simulink model "GVCU_HIL_simscape"  (R2026a)
settings: Solver=ode3  StartTime=0  StopTime=10  FixedStep=0.001
model workspace (MAT data in the model file):
  CANoelibParameters : object (value not decoded)
values from neighbouring files (symbols this model uses):
  acc_pedal_data = pedal_data.accelerator_pedal_position_t0    [Init_Simscape_main.m]
  acc_pedal_time = pedal_data.t0    [Init_Simscape_main.m]
  brk_pedal_data = brake_pedal_data.shared_brakes_drvrBrkPedlPerc_t0    [Init_Simscape_main.m]
  brk_pedal_time = brake_pedal_data.t0    [Init_Simscape_main.m]
  cycle_len = zeros(1, num_cycles)    [Init_Simscape_main.m]
  cycle_speed_matrix = zeros(max_cycle_len, num_cycles)    [Init_Simscape_main.m]
  cycle_time_matrix = zeros(max_cycle_len, num_cycles)    [Init_Simscape_main.m]
  veh_speed_data = speed_data.shared_dynamicsVso_vehVelLgt_t0    [Init_Simscape_main.m]
  veh_speed_time = speed_data.t0    [Init_Simscape_main.m]
undefined symbols (not defined in the file or in its folder): Active, aero, AuxActive, bat, brake, config, environment, FL, FL_prs_voltage, FR, FR_prs_voltage, front, pos, powertrain, rear, RL, RL_prs_voltage, RR, RR_prs_voltage, tir, veh, VGetRawValueFlag, Voltage, VT2816_1_Ch1, VT2816_1_Ch2, VT2816_1_Ch3, VT2816_1_Ch4, VT2816_3_Ch13, VT2816_3_Ch14, VT7101_1_Out2, VTS, X, Y, Z
libraries: sm_lib x358, fl_lib x272, nesl_utility x193, canoelib x127, sdl_lib x36, autolibsharedcoupling x21, autolibcoupling x9, slpidlib x7, simulink x3, autolibshareddiff x3, autolibshared x3, autolibutils x1
(part 9 of 17)

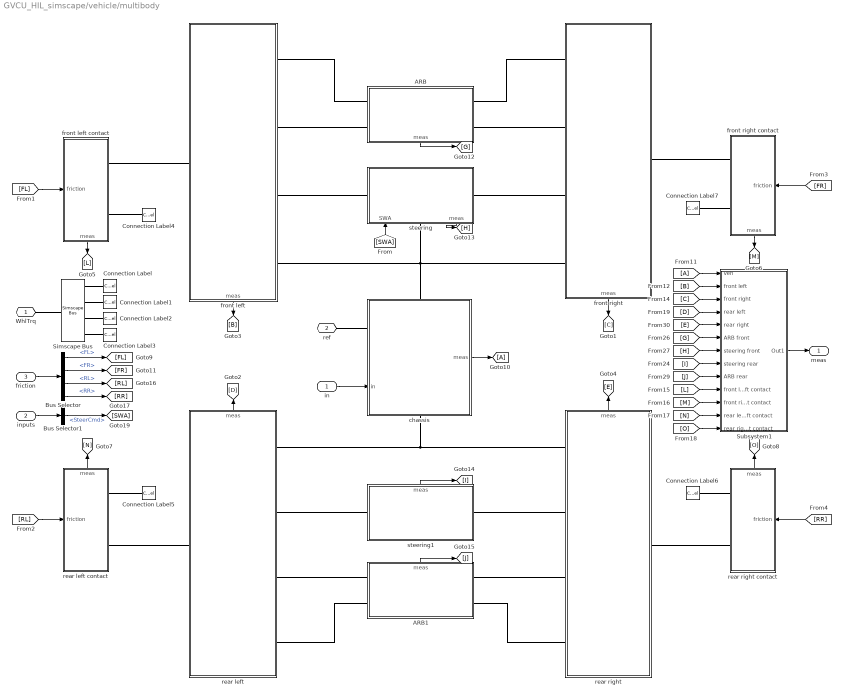
== system GVCU_HIL_simscape/vehicle/multibody ==
  in : Inport
  inputs : Inport  Port=2
  friction : Inport  Port=3
  ARB : Subsystem
      settings: PortSchema="{\"entries\":[{\"content\":{\"sides\":[{\"content\":{\"connectorIds\":[\"LConn1\",\"LConn2\"]},\"type\":\"ConnectorPlacement.EquallySpacedRectSide\",\"uuid\":\"44b83d78-7117-4f50-a128-c40c6db0e005\"},{\"content\":{\"connectorIds\":[\"RConn1\",\"RConn2\"],\"side\":\"RIGHT\"},\"type\":\"ConnectorPlacement.EquallySpacedRectSide\",\"uuid\":\"dcc56467-eb52-44b2-a421-ed24436307ce\"},{\"content\":{\"side\":\"TOP\"},\"type\":\"ConnectorPlacement.EquallySpacedRectSide\",\"uuid\":\"66a42ba5-e53f-479b-a6ea-7e29dc8adaf6\"},{\"content\":{\"connectorIds\":[\"Out1\"],\"side\":\"BOTTOM\"},\"type\":\"ConnectorPlacement.EquallySpacedRectSide\",\"uuid\":\"e20d4be4-d4bb-4d26-9635-b654396fd56f\"}]},\"type\":\"ConnectorPlacement.EquallySpacedConnector\",\"uuid\":\"7509cb20-f578-40f8-ba61-999a8824cfe4\"}],\"packageUris\":[\"http://schema.mathworks.com/mf0/Connector/R2020b\"],\"version\":\"1.0\"}"
  ARB1 : Subsystem
      settings: PortSchema="{\"entries\":[{\"content\":{\"sides\":[{\"content\":{\"connectorIds\":[\"LConn1\",\"LConn2\"]},\"type\":\"ConnectorPlacement.EquallySpacedRectSide\",\"uuid\":\"44b83d78-7117-4f50-a128-c40c6db0e005\"},{\"content\":{\"connectorIds\":[\"RConn1\",\"RConn2\"],\"side\":\"RIGHT\"},\"type\":\"ConnectorPlacement.EquallySpacedRectSide\",\"uuid\":\"dcc56467-eb52-44b2-a421-ed24436307ce\"},{\"content\":{\"connectorIds\":[\"Out1\"],\"side\":\"TOP\"},\"type\":\"ConnectorPlacement.EquallySpacedRectSide\",\"uuid\":\"66a42ba5-e53f-479b-a6ea-7e29dc8adaf6\"}]},\"type\":\"ConnectorPlacement.EquallySpacedConnector\",\"uuid\":\"7509cb20-f578-40f8-ba61-999a8824cfe4\"}],\"packageUris\":[\"http://schema.mathworks.com/mf0/Connector/R2020b\"],\"version\":\"1.0\"}"
  Bus Selector : BusSelector  OutputSignals=FL,FR,RL,RR
  Bus Selector1 : BusSelector  OutputSignals=SteerCmd
  Connection Label : ConnectionLabel  Label=FL
  Connection Label1 : ConnectionLabel  Label=FR
  Connection Label2 : ConnectionLabel  Label=RL
  Connection Label3 : ConnectionLabel  Label=RR
  Connection Label4 : ConnectionLabel  Label=FL
  Connection Label5 : ConnectionLabel  Label=RL
  Connection Label6 : ConnectionLabel  Label=RR
  Connection Label7 : ConnectionLabel  Label=FR
  From11 : From
  Goto10 : Goto
  Simscape Bus : SimscapeBus  HierarchyStrings=FL;FR;RL;RR
  Subsystem1 : Subsystem
  chassis : Subsystem
      settings: PortSchema="{\"entries\":[{\"content\":{\"sides\":[{\"content\":{\"connectorIds\":[\"LConn1\",\"In1\"]},\"type\":\"ConnectorPlacement.EquallySpacedRectSide\",\"uuid\":\"c24a0a87-e96f-44b7-bb9d-4d54604155f4\"},{\"content\":{\"connectorIds\":[\"Out1\"],\"side\":\"RIGHT\"},\"type\":\"ConnectorPlacement.EquallySpacedRectSide\",\"uuid\":\"a7cb0370-4bed-448c-a8ed-597510355169\"},{\"content\":{\"connectorIds\":[\"LConn2\"],\"side\":\"TOP\"},\"type\":\"ConnectorPlacement.EquallySpacedRectSide\",\"uuid\":\"f3c52e5d-562f-4591-a778-2d78a942b9f8\"},{\"content\":{\"connectorIds\":[\"RConn1\"],\"side\":\"BOTTOM\"},\"type\":\"ConnectorPlacement.EquallySpacedRectSide\",\"uuid\":\"7ef3619e-825e-48e3-8fdb-b0e1b2ee4c3a\"}]},\"type\":\"ConnectorPlacement.EquallySpacedConnector\",\"uuid\":\"67b61cb1-688b-4fcf-aa15-016bbf82641a\"}],\"packageUris\":[\"http://schema.mathworks.com/mf0/Connector/R2020b\"],\"version\":\"1.0\"}"
  front left : Subsystem
      settings: PortSchema="{\"entries\":[{\"content\":{\"sides\":[{\"content\":{\"connectorIds\":[\"LConn1\"]},\"type\":\"ConnectorPlacement.EquallySpacedRectSide\",\"uuid\":\"19de201b-0d55-468b-9ae9-f040ed0ebaa1\"},{\"content\":{\"connectorIds\":[\"RConn1\",\"RConn2\",\"RConn3\",\"RConn4\"],\"side\":\"RIGHT\"},\"type\":\"ConnectorPlacement.EquallySpacedRectSide\",\"uuid\":\"0a313072-8af5-469b-b8e4-48bb708ad821\"},{\"content\":{\"side\":\"TOP\"},\"type\":\"ConnectorPlacement.EquallySpacedRectSide\",\"uuid\":\"5fa73a83-add4-41d1-8bf2-6e1c7ef44456\"},{\"content\":{\"connectorIds\":[\"Out1\"],\"side\":\"BOTTOM\"},\"type\":\"ConnectorPlacement.EquallySpacedRectSide\",\"uuid\":\"99aac4ff-0e91-4277-96be-b0211bbbd05e\"}]},\"type\":\"ConnectorPlacement.EquallySpacedConnector\",\"uuid\":\"0106dc40-6661-4c74-95ab-8e6f8c5e0ff4\"}],\"packageUris\":[\"http://schema.mathworks.com/mf0/Connector/R2020b\"],\"version\":\"1.0\"}"
  front left contact : Subsystem
      settings: PortSchema="{\"entries\":[{\"content\":{\"sides\":[{\"content\":{\"connectorIds\":[\"In1\"]},\"type\":\"ConnectorPlacement.EquallySpacedRectSide\",\"uuid\":\"10158845-5afa-461c-a22d-1b912d59afd1\"},{\"content\":{\"connectorIds\":[\"RConn1\",\"RConn2\"],\"side\":\"RIGHT\"},\"type\":\"ConnectorPlacement.EquallySpacedRectSide\",\"uuid\":\"d8f36145-e6de-4ff7-929e-d1b9d10fe783\"},{\"content\":{\"side\":\"TOP\"},\"type\":\"ConnectorPlacement.EquallySpacedRectSide\",\"uuid\":\"7f3dfbca-e54d-431a-ba74-3f88cb4ee578\"},{\"content\":{\"connectorIds\":[\"Out1\"],\"side\":\"BOTTOM\"},\"type\":\"ConnectorPlacement.EquallySpacedRectSide\",\"uuid\":\"2d75498b-d206-48f5-8aff-45cacbfc615a\"}]},\"type\":\"ConnectorPlacement.EquallySpacedConnector\",\"uuid\":\"094a29d2-4f54-4ab7-b7e4-df405ec9cb17\"}],\"packageUris\":[\"http://schema.mathworks.com/mf0/Connector/R2020b\"],\"version\":\"1.0\"}"
  front right : Subsystem
      settings: PortSchema="{\"entries\":[{\"content\":{\"sides\":[{\"content\":{\"connectorIds\":[\"LConn1\",\"LConn2\",\"LConn3\",\"LConn4\"]},\"type\":\"ConnectorPlacement.EquallySpacedRectSide\",\"uuid\":\"1e088fd9-3d93-474e-8fe9-197185a633cf\"},{\"content\":{\"connectorIds\":[\"RConn1\"],\"side\":\"RIGHT\"},\"type\":\"ConnectorPlacement.EquallySpacedRectSide\",\"uuid\":\"782d0377-23b5-4dfd-8ac7-d3568aae0714\"},{\"content\":{\"side\":\"TOP\"},\"type\":\"ConnectorPlacement.EquallySpacedRectSide\",\"uuid\":\"3962e876-5f8e-408b-8e08-ce800b05363f\"},{\"content\":{\"connectorIds\":[\"Out1\"],\"side\":\"BOTTOM\"},\"type\":\"ConnectorPlacement.EquallySpacedRectSide\",\"uuid\":\"745efcfe-4536-4516-bf5a-c30453ee72e3\"}]},\"type\":\"ConnectorPlacement.EquallySpacedConnector\",\"uuid\":\"ffd119f6-ad19-4d62-b08f-fd8048e53da0\"}],\"packageUris\":[\"http://schema.mathworks.com/mf0/Connector/R2020b\"],\"version\":\"1.0\"}"
  front right contact : Subsystem
      settings: PortSchema="{\"entries\":[{\"content\":{\"sides\":[{\"content\":{\"connectorIds\":[\"In1\"]},\"type\":\"ConnectorPlacement.EquallySpacedRectSide\",\"uuid\":\"366ed39c-e506-485f-aedc-43f3a008ee89\"},{\"content\":{\"connectorIds\":[\"RConn1\",\"RConn2\"],\"side\":\"RIGHT\"},\"type\":\"ConnectorPlacement.EquallySpacedRectSide\",\"uuid\":\"70a828f7-7299-4f1a-95a3-d8e7b8390954\"},{\"content\":{\"connectorIds\":[\"Out1\"],\"side\":\"TOP\"},\"type\":\"ConnectorPlacement.EquallySpacedRectSide\",\"uuid\":\"0ab3354d-2824-40db-aebc-c093b7d793d8\"}]},\"type\":\"ConnectorPlacement.EquallySpacedConnector\",\"uuid\":\"4490982e-7f0c-4997-9546-ef978a19b2a8\"}],\"packageUris\":[\"http://schema.mathworks.com/mf0/Connector/R2020b\"],\"version\":\"1.0\"}"
  rear left : Subsystem
      settings: PortSchema="{\"entries\":[{\"content\":{\"sides\":[{\"content\":{\"connectorIds\":[\"LConn1\"]},\"type\":\"ConnectorPlacement.EquallySpacedRectSide\",\"uuid\":\"99636ad2-3001-422b-8269-7f0afa543239\"},{\"content\":{\"connectorIds\":[\"RConn1\",\"RConn2\",\"RConn3\",\"RConn4\"],\"side\":\"RIGHT\"},\"type\":\"ConnectorPlacement.EquallySpacedRectSide\",\"uuid\":\"6caf7980-c550-4646-898e-a2e6d571860b\"},{\"content\":{\"connectorIds\":[\"Out1\"],\"side\":\"TOP\"},\"type\":\"ConnectorPlacement.EquallySpacedRectSide\",\"uuid\":\"53eccbec-cba9-4e03-a09a-c4bd8c593235\"},{\"content\":{\"side\":\"BOTTOM\"},\"type\":\"ConnectorPlacement.EquallySpacedRectSide\",\"uuid\":\"e369446d-0d30-47ff-9006-d12c8ecdecf9\"}]},\"type\":\"ConnectorPlacement.EquallySpacedConnector\",\"uuid\":\"292a83a5-3a3e-4909-8366-ad11964dade1\"}],\"packageUris\":[\"http://schema.mathworks.com/mf0/Connector/R2020b\"],\"version\":\"1.0\"}"
  rear left contact : Subsystem
      settings: PortSchema="{\"entries\":[{\"content\":{\"sides\":[{\"content\":{\"connectorIds\":[\"In1\"]},\"type\":\"ConnectorPlacement.EquallySpacedRectSide\",\"uuid\":\"10158845-5afa-461c-a22d-1b912d59afd1\"},{\"content\":{\"connectorIds\":[\"RConn1\",\"RConn2\"],\"side\":\"RIGHT\"},\"type\":\"ConnectorPlacement.EquallySpacedRectSide\",\"uuid\":\"d8f36145-e6de-4ff7-929e-d1b9d10fe783\"},{\"content\":{\"connectorIds\":[\"Out1\"],\"side\":\"TOP\"},\"type\":\"ConnectorPlacement.EquallySpacedRectSide\",\"uuid\":\"7f3dfbca-e54d-431a-ba74-3f88cb4ee578\"}]},\"type\":\"ConnectorPlacement.EquallySpacedConnector\",\"uuid\":\"094a29d2-4f54-4ab7-b7e4-df405ec9cb17\"}],\"packageUris\":[\"http://schema.mathworks.com/mf0/Connector/R2020b\"],\"version\":\"1.0\"}"
  rear right : Subsystem
      settings: PortSchema="{\"entries\":[{\"content\":{\"sides\":[{\"content\":{\"connectorIds\":[\"LConn1\",\"LConn2\",\"LConn3\",\"LConn4\"]},\"type\":\"ConnectorPlacement.EquallySpacedRectSide\",\"uuid\":\"97554ec7-9fc3-491f-8a72-eaeb56dc13e3\"},{\"content\":{\"connectorIds\":[\"RConn1\"],\"side\":\"RIGHT\"},\"type\":\"ConnectorPlacement.EquallySpacedRectSide\",\"uuid\":\"01e3ceb2-8653-48cc-8018-c9fa0765a906\"},{\"content\":{\"connectorIds\":[\"Out1\"],\"side\":\"TOP\"},\"type\":\"ConnectorPlacement.EquallySpacedRectSide\",\"uuid\":\"f66f365d-d7f1-473b-ac81-c34d456abf41\"}]},\"type\":\"ConnectorPlacement.EquallySpacedConnector\",\"uuid\":\"3daf5b58-372f-4a47-a824-31f905f9d0f6\"}],\"packageUris\":[\"http://schema.mathworks.com/mf0/Connector/R2020b\"],\"version\":\"1.0\"}"
  rear right contact : Subsystem
      settings: PortSchema="{\"entries\":[{\"content\":{\"sides\":[{\"content\":{\"connectorIds\":[\"LConn1\",\"LConn2\"]},\"type\":\"ConnectorPlacement.EquallySpacedRectSide\",\"uuid\":\"50c969ea-b4f9-4e95-a8d7-0439ee002930\"},{\"content\":{\"connectorIds\":[\"In1\"],\"side\":\"RIGHT\"},\"type\":\"ConnectorPlacement.EquallySpacedRectSide\",\"uuid\":\"21bba6f4-d340-4ba8-8ff8-cca6003000cc\"},{\"content\":{\"connectorIds\":[\"Out1\"],\"side\":\"TOP\"},\"type\":\"ConnectorPlacement.EquallySpacedRectSide\",\"uuid\":\"17e17638-e1d3-4216-888f-e3f212538333\"}]},\"type\":\"ConnectorPlacement.EquallySpacedConnector\",\"uuid\":\"e91be55c-c97e-45e3-9316-75c991eef38b\"}],\"packageUris\":[\"http://schema.mathworks.com/mf0/Connector/R2020b\"],\"version\":\"1.0\"}"
  steering : Subsystem
      settings: PortSchema="{\"entries\":[{\"content\":{\"sides\":[{\"content\":{\"connectorIds\":[\"LConn1\"]},\"type\":\"ConnectorPlacement.EquallySpacedRectSide\",\"uuid\":\"8d82ea5c-1bae-45fe-ac82-53123a9b3f5e\"},{\"content\":{\"connectorIds\":[\"RConn1\"],\"side\":\"RIGHT\"},\"type\":\"ConnectorPlacement.EquallySpacedRectSide\",\"uuid\":\"e2db56e2-8468-453e-a935-2b5d90d5c02e\"},{\"content\":{\"side\":\"TOP\"},\"type\":\"ConnectorPlacement.EquallySpacedRectSide\",\"uuid\":\"66f010a1-1264-4266-a794-e542ee8c9be7\"},{\"content\":{\"connectorIds\":[\"In1\",\"RConn2\",\"Out1\"],\"side\":\"BOTTOM\"},\"type\":\"ConnectorPlacement.EquallySpacedRectSide\",\"uuid\":\"2ab87368-c822-4cdb-a3b2-bb1f2e0cbe7f\"}]},\"type\":\"ConnectorPlacement.EquallySpacedConnector\",\"uuid\":\"219c3897-806d-4045-90e2-26bf99ed85a1\"}],\"packageUris\":[\"http://schema.mathworks.com/mf0/Connector/R2020b\"],\"version\":\"1.0\"}"
  steering1 : Subsystem
      settings: PortSchema="{\"entries\":[{\"content\":{\"sides\":[{\"content\":{\"connectorIds\":[\"LConn1\"]},\"type\":\"ConnectorPlacement.EquallySpacedRectSide\",\"uuid\":\"fb5a7c7c-1f71-468f-8e2b-293f168c4d3f\"},{\"content\":{\"connectorIds\":[\"RConn1\"],\"side\":\"RIGHT\"},\"type\":\"ConnectorPlacement.EquallySpacedRectSide\",\"uuid\":\"5b9e4945-a95c-4a22-ad9b-f4b0b8937fba\"},{\"content\":{\"connectorIds\":[\"Out1\"],\"side\":\"TOP\"},\"type\":\"ConnectorPlacement.EquallySpacedRectSide\",\"uuid\":\"934bce12-3f30-409e-b265-a8a1cc310c4a\"}]},\"type\":\"ConnectorPlacement.EquallySpacedConnector\",\"uuid\":\"f5a21e72-9783-4a4e-b870-1cf7e777535b\"}],\"packageUris\":[\"http://schema.mathworks.com/mf0/Connector/R2020b\"],\"version\":\"1.0\"}"
  WhlTrq : PMIOPort  Side=Left
  ref : PMIOPort  Port=2  Side=Left
  meas : Outport
  wires:
  [SWA] -> steering/1(SWA)
  front left/1(meas) -> [B]
  rear right contact/1(meas) -> [O]
  rear left contact/1(meas) -> [N]
  front left contact/1(meas) -> [L]
  front right/1(meas) -> [C]
  rear left/1(meas) -> [D]
  front right contact/1(meas) -> [M]
  chassis/1(meas) -> Goto10/1
  rear right/1(meas) -> [E]
  Bus Selector1/1 -> [SWA]  "<SteerCmd>"
  inputs/1 -> Bus Selector1/1
  ARB/1(meas) -> [G]
  steering/1(meas) -> [H]
  steering1/1(meas) -> [I]
  ARB1/1(meas) -> [J]
  [B] -> Subsystem1/2(front left)
  [L] -> Subsystem1/10(front left contact)
  [C] -> Subsystem1/3(front right)
  [M] -> Subsystem1/11(front right contact)
  [G] -> Subsystem1/6(ARB front)
  [H] -> Subsystem1/7(steering front)
  [D] -> Subsystem1/4(rear left)
  [N] -> Subsystem1/12(rear left contact)
  [E] -> Subsystem1/5(rear right)
  [O] -> Subsystem1/13(rear right contact)
  [I] -> Subsystem1/8(steering rear)
  [J] -> Subsystem1/9(ARB rear)
  From11/1 -> Subsystem1/1(veh)
  Subsystem1/1(Out1) -> meas/1
  in/1 -> chassis/1(in)
  friction/1 -> Bus Selector/1
  Bus Selector/1 -> [FL]  "<FL>"
  Bus Selector/2 -> [FR]  "<FR>"
  Bus Selector/3 -> [RL]  "<RL>"
  Bus Selector/4 -> [RR]  "<RR>"
  [FL] -> front left contact/1(friction)
  [RL] -> rear left contact/1(friction)
  [FR] -> front right contact/1(friction)
  [RR] -> rear right contact/1(friction)
  connections:
  Connection Label7/LConn1 -- front right contact/RConn1
  ref/RConn1 -- chassis/LConn1
  ARB1/RConn2 -- rear right/LConn4
  rear left/RConn1 -- chassis/RConn1 -- rear right/LConn1
  front left/RConn4 -- steering/RConn2 -- front right/LConn4 -- chassis/LConn2
  Connection Label4/LConn1 -- front left contact/RConn2
  ARB/RConn1 -- front right/LConn1
  front left/RConn2 -- ARB/LConn2
  ARB/RConn2 -- front right/LConn2
  front right/RConn1 -- front right contact/RConn2
  steering/RConn1 -- front right/LConn3
  front left/RConn1 -- ARB/LConn1
  front left contact/RConn1 -- front left/LConn1
  rear right contact/LConn2 -- rear right/RConn1
  steering1/LConn1 -- rear left/RConn2
  rear left/RConn4 -- ARB1/LConn2
  rear left/RConn3 -- ARB1/LConn1
  rear right/LConn2 -- steering1/RConn1
  ARB1/RConn1 -- rear right/LConn3
  rear left contact/RConn2 -- rear left/LConn1
  Connection Label6/LConn1 -- rear right contact/LConn1
  steering/LConn1 -- front left/RConn3
  Connection Label5/LConn1 -- rear left contact/RConn1
  Simscape Bus/RConn1 -- WhlTrq/RConn1
  Connection Label/LConn1 -- Simscape Bus/LConn1
  Simscape Bus/LConn2 -- Connection Label1/LConn1
  Simscape Bus/LConn3 -- Connection Label2/LConn1
  Simscape Bus/LConn4 -- Connection Label3/LConn1

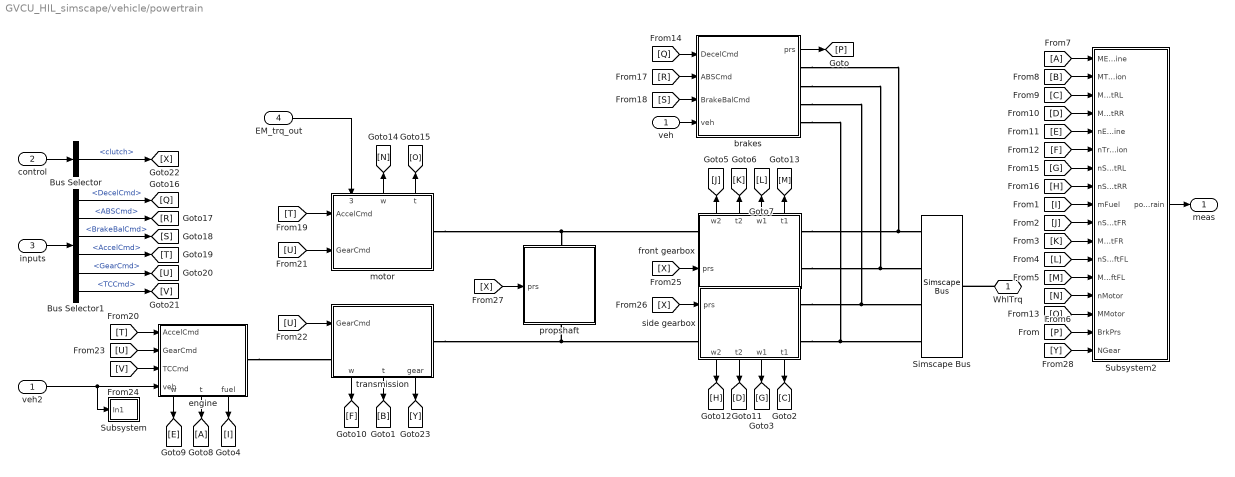
== system GVCU_HIL_simscape/vehicle/powertrain ==
  veh : Inport
  control : Inport  Port=2
  inputs : Inport  Port=3
  EM_trq_out : Inport  Port=4
  Bus Selector : BusSelector  OutputSignals=clutch
  Bus Selector1 : BusSelector  OutputSignals=DecelCmd,ABSCmd,BrakeBalCmd,AccelCmd,GearCmd,TCCmd
  From7 : From
  Goto8 : Goto
  Simscape Bus : SimscapeBus  HierarchyStrings=FL;FR;RL;RR
  Subsystem : Subsystem
  Subsystem2 : Subsystem
  brakes : Subsystem
  engine : Subsystem
      settings: PortSchema="{\"entries\":[{\"content\":{\"sides\":[{\"content\":{\"connectorIds\":[\"In1\",\"In2\",\"In3\",\"In4\"]},\"type\":\"ConnectorPlacement.EquallySpacedRectSide\",\"uuid\":\"a78e3356-1921-4efa-86ee-ec197aedbb96\"},{\"content\":{\"connectorIds\":[\"RConn1\"],\"side\":\"RIGHT\"},\"type\":\"ConnectorPlacement.EquallySpacedRectSide\",\"uuid\":\"41546e87-53dd-47be-ad0a-44218c6e7147\"},{\"content\":{\"side\":\"TOP\"},\"type\":\"ConnectorPlacement.EquallySpacedRectSide\",\"uuid\":\"0868fe6a-0ce7-41c0-87b1-c24c29d5bf2c\"},{\"content\":{\"connectorIds\":[\"Out1\",\"Out2\",\"Out3\"],\"side\":\"BOTTOM\"},\"type\":\"ConnectorPlacement.EquallySpacedRectSide\",\"uuid\":\"e86847d3-d00d-4616-b427-8230020483c2\"}]},\"type\":\"ConnectorPlacement.EquallySpacedConnector\",\"uuid\":\"338a52b8-b908-4274-bc1a-a3eae903fb18\"}],\"packageUris\":[\"http://schema.mathworks.com/mf0/Connector/R2020b\"],\"version\":\"1.0\"}"
  front gearbox : Subsystem
      settings: PortSchema="{\"entries\":[{\"content\":{\"sides\":[{\"content\":{\"connectorIds\":[\"LConn1\",\"In1\"]},\"type\":\"ConnectorPlacement.EquallySpacedRectSide\",\"uuid\":\"4b5bd540-f981-403d-a3c0-21cea5792707\"},{\"content\":{\"connectorIds\":[\"RConn1\",\"RConn2\"],\"side\":\"RIGHT\"},\"type\":\"ConnectorPlacement.EquallySpacedRectSide\",\"uuid\":\"db8e6c45-4440-4c46-8526-795a478301ab\"},{\"content\":{\"connectorIds\":[\"Out1\",\"Out2\",\"Out3\",\"Out4\"],\"side\":\"TOP\"},\"type\":\"ConnectorPlacement.EquallySpacedRectSide\",\"uuid\":\"3c4f3c49-5b91-4a57-ad94-4436adb36465\"}]},\"type\":\"ConnectorPlacement.EquallySpacedConnector\",\"uuid\":\"873cdc70-bb12-4c47-8236-9ecaebb66c28\"}],\"packageUris\":[\"http://schema.mathworks.com/mf0/Connector/R2020b\"],\"version\":\"1.0\"}"
  motor : Subsystem
      settings: PortSchema="{\"entries\":[{\"content\":{\"sides\":[{\"content\":{\"connectorIds\":[\"In1\",\"In2\"]},\"type\":\"ConnectorPlacement.EquallySpacedRectSide\",\"uuid\":\"8872ef77-aef5-44ab-bd09-c386537b6db6\"},{\"content\":{\"connectorIds\":[\"RConn1\"],\"side\":\"RIGHT\"},\"type\":\"ConnectorPlacement.EquallySpacedRectSide\",\"uuid\":\"8e814109-7cc3-4dbb-af0e-0bb3c3af015b\"},{\"content\":{\"connectorIds\":[\"In3\",\"Out1\",\"Out2\"],\"side\":\"TOP\"},\"type\":\"ConnectorPlacement.EquallySpacedRectSide\",\"uuid\":\"d6bbb977-d9f2-49ac-8838-af9f0d5a07e1\"}]},\"type\":\"ConnectorPlacement.EquallySpacedConnector\",\"uuid\":\"ff2df442-a81d-42d1-91a4-930a8e06f842\"}],\"packageUris\":[\"http://schema.mathworks.com/mf0/Connector/R2020b\"],\"version\":\"1.0\"}"
  propshaft : Subsystem
      settings: PortSchema="{\"entries\":[{\"content\":{\"sides\":[{\"content\":{\"connectorIds\":[\"In1\"]},\"type\":\"ConnectorPlacement.EquallySpacedRectSide\",\"uuid\":\"d74c70ba-453f-40cc-b257-82be2cfc77c8\"},{\"content\":{\"side\":\"RIGHT\"},\"type\":\"ConnectorPlacement.EquallySpacedRectSide\",\"uuid\":\"3ad33456-fba7-46bf-9dae-3669e8d1c7bf\"},{\"content\":{\"connectorIds\":[\"LConn1\"],\"side\":\"TOP\"},\"type\":\"ConnectorPlacement.EquallySpacedRectSide\",\"uuid\":\"e56339ea-fe76-4a6c-8c1f-8950ec15449d\"},{\"content\":{\"connectorIds\":[\"RConn1\"],\"side\":\"BOTTOM\"},\"type\":\"ConnectorPlacement.EquallySpacedRectSide\",\"uuid\":\"99006158-d2e6-44ab-b5b9-386e2116889a\"}]},\"type\":\"ConnectorPlacement.EquallySpacedConnector\",\"uuid\":\"1e2408ea-7505-408f-9d6e-80dc061e9f6e\"}],\"packageUris\":[\"http://schema.mathworks.com/mf0/Connector/R2020b\"],\"version\":\"1.0\"}"
  side gearbox : Subsystem
      settings: PortSchema="{\"entries\":[{\"content\":{\"sides\":[{\"content\":{\"connectorIds\":[\"In1\",\"LConn1\"]},\"type\":\"ConnectorPlacement.EquallySpacedRectSide\",\"uuid\":\"8c94453b-f679-4642-95d3-f9d99a2c2408\"},{\"content\":{\"connectorIds\":[\"RConn1\",\"RConn2\"],\"side\":\"RIGHT\"},\"type\":\"ConnectorPlacement.EquallySpacedRectSide\",\"uuid\":\"3bcbea54-e5b0-4650-b782-00c18ea383a7\"},{\"content\":{\"side\":\"TOP\"},\"type\":\"ConnectorPlacement.EquallySpacedRectSide\",\"uuid\":\"707a6b03-da98-480f-b93c-3d32e5658bd5\"},{\"content\":{\"connectorIds\":[\"Out1\",\"Out2\",\"Out3\",\"Out4\"],\"side\":\"BOTTOM\"},\"type\":\"ConnectorPlacement.EquallySpacedRectSide\",\"uuid\":\"a2021d0b-6ca2-49e7-9b1d-c01e0bfdef0d\"}]},\"type\":\"ConnectorPlacement.EquallySpacedConnector\",\"uuid\":\"d21a57c1-8b78-49d8-b9d2-27b607922f0d\"}],\"packageUris\":[\"http://schema.mathworks.com/mf0/Connector/R2020b\"],\"version\":\"1.0\"}"
  transmission : Subsystem
      settings: PortSchema="{\"entries\":[{\"content\":{\"sides\":[{\"content\":{\"connectorIds\":[\"In1\",\"LConn1\"]},\"type\":\"ConnectorPlacement.EquallySpacedRectSide\",\"uuid\":\"86e8cea5-b07c-40dd-bb6b-836fb2a21237\"},{\"content\":{\"connectorIds\":[\"RConn1\"],\"side\":\"RIGHT\"},\"type\":\"ConnectorPlacement.EquallySpacedRectSide\",\"uuid\":\"59522f78-d2d1-447e-be1e-cdc3e72ed8cb\"},{\"content\":{\"side\":\"TOP\"},\"type\":\"ConnectorPlacement.EquallySpacedRectSide\",\"uuid\":\"b992db60-f6d2-4879-b98d-54a12f763f72\"},{\"content\":{\"connectorIds\":[\"Out1\",\"Out2\",\"Out3\"],\"side\":\"BOTTOM\"},\"type\":\"ConnectorPlacement.EquallySpacedRectSide\",\"uuid\":\"d7b1bd10-aa14-42f4-8993-c98a02d1ca10\"}]},\"type\":\"ConnectorPlacement.EquallySpacedConnector\",\"uuid\":\"b24a2d83-8980-4644-9416-64d6e84609ca\"}],\"packageUris\":[\"http://schema.mathworks.com/mf0/Connector/R2020b\"],\"version\":\"1.0\"}"
  veh2 : InportShadow
  WhlTrq : PMIOPort  Side=Right
  meas : Outport
  wires:
  Bus Selector1/5 -> [U]  "<GearCmd>"
  inputs/1 -> Bus Selector1/1
  Bus Selector1/1 -> [Q]  "<DecelCmd>"
  Bus Selector1/4 -> [T]  "<AccelCmd>"
  engine/2(t) -> Goto8/1
  engine/1(w) -> [E]
  transmission/2(t) -> [B]
  transmission/1(w) -> [F]
  side gearbox/4(t1) -> [C]
  side gearbox/3(w1) -> [G]
  side gearbox/2(t2) -> [D]
  side gearbox/1(w2) -> [H]
  Bus Selector1/3 -> [S]  "<BrakeBalCmd>"
  veh/1 -> brakes/4(veh)
  Bus Selector1/2 -> [R]  "<ABSCmd>"
  Bus Selector1/6 -> [V]  "<TCCmd>"
  veh2/1 -> Subsystem/1(In1), engine/4(veh)
  From7/1 -> Subsystem2/1(MEngine)
  [B] -> Subsystem2/2(MTransmission)
  [C] -> Subsystem2/3(MSideShaftRL)
  [D] -> Subsystem2/4(MSideShaftRR)
  [E] -> Subsystem2/5(nEngine)
  [F] -> Subsystem2/6(nTransmission)
  [G] -> Subsystem2/7(nSideShaftRL)
  [H] -> Subsystem2/8(nSideShaftRR)
  Subsystem2/1(powertrain) -> meas/1
  engine/3(fuel) -> [I]
  [I] -> Subsystem2/9(mFuel)
  front gearbox/1(w2) -> [J]
  front gearbox/2(t2) -> [K]
  front gearbox/3(w1) -> [L]
  front gearbox/4(t1) -> [M]
  [M] -> Subsystem2/13(MSideShaftFL)
  [L] -> Subsystem2/12(nSideShaftFL)
  [K] -> Subsystem2/11(MSideShaftFR)
  [J] -> Subsystem2/10(nSIdeShaftFR)
  motor/1(w) -> [N]
  motor/2(t) -> [O]
  [N] -> Subsystem2/14(nMotor)
  [O] -> Subsystem2/15(MMotor)
  brakes/1(prs) -> [P]
  [P] -> Subsystem2/16(BrkPrs)
  [Q] -> brakes/1(DecelCmd)
  [R] -> brakes/2(ABSCmd)
  [S] -> brakes/3(BrakeBalCmd)
  [T] -> motor/1(AccelCmd)
  [T] -> engine/1(AccelCmd)
  [U] -> motor/2(GearCmd)
  [U] -> transmission/1(GearCmd)
  [U] -> engine/2(GearCmd)
  [V] -> engine/3(TCCmd)
  [X] -> front gearbox/1(prs)
  [X] -> side gearbox/1(prs)
  [X] -> propshaft/1(prs)
  control/1 -> Bus Selector/1
  Bus Selector/1 -> [X]  "<clutch>"
  transmission/3(gear) -> [Y]
  [Y] -> Subsystem2/17(NGear)
  EM_trq_out/1 -> motor/3(EM_trq_out)
  connections:
  brakes/RConn1 -- front gearbox/RConn1 -- Simscape Bus/LConn1
  brakes/RConn2 -- front gearbox/RConn2 -- Simscape Bus/LConn2
  engine/RConn1 -- transmission/LConn1
  side gearbox/RConn2 -- brakes/RConn4 -- Simscape Bus/LConn4
  side gearbox/RConn1 -- brakes/RConn3 -- Simscape Bus/LConn3
  transmission/RConn1 -- propshaft/RConn1 -- side gearbox/LConn1
  WhlTrq/RConn1 -- Simscape Bus/RConn1
  motor/RConn1 -- propshaft/LConn1 -- front gearbox/LConn1

== system GVCU_HIL_simscape/Driver/Driver/Dec_controller ==
  Vel_ref : Inport
  Vel_fdk : Inport  Port=2
  PI Controller : slpidlib/PID Controller  Controller=PI  Form=Parallel  TimeDomain=Discrete-time  UseExternalTs=off  SampleTime=-1  IntegratorMethod=Forward Euler  FilterMethod=Forward Euler  ControllerParametersSource=internal  P=1  I=1  UseKiTs=on  D=0  UseExternalDerivativeSource=off  N=100  UseFilter=on  TunerSelectOption=Transfer Function Based (PID Tuner App)  InitialConditionSource=internal  InitialConditionForIntegrator=0  InitialConditionForFilter=0  DifferentiatorICPrevScaledInput=0  ExternalReset=level  TrackingMode=off  Kt=1  LimitOutput=on  SatLimitsSource=internal  UpperSaturationLimit=50  LowerSaturationLimit=0  LinearizeAsGain=on  AntiWindupMode=clamping  Kb=1  LimitIntegrator=off  UpperIntegratorSaturationLimit=inf  LowerIntegratorSaturationLimit=-inf  RndMeth=Simplest  POutMin=[]  POutMax=[]  IOutMin=[]  IOutMax=[]  DOutMin=[]  DOutMax=[]  NOutMin=[]  NOutMax=[]  SumOutMin=[]  SumOutMax=[]  SaturationOutDataTypeStr=Inherit: Inherit via back propagation  SaturationOutMin=[]  SaturationOutMax=[]  PParamMin=[]  PParamMax=[]  IParamMin=[]  IParamMax=[]  DParamMin=[]  DParamMax=[]  NParamMin=[]  NParamMax=[]  KbParamMin=[]  KbParamMax=[]  KtParamMin=[]  KtParamMax=[]  KbOutMin=[]  KbOutMax=[]  KtOutMin=[]  KtOutMax=[]  IntegratorOutMin=[]  IntegratorOutMax=[]  FilterOutMin=[]  FilterOutMax=[]  SumI1OutMin=[]  SumI1OutMax=[]  SumI2OutMin=[]  SumI2OutMax=[]  SumI3OutMin=[]  SumI3OutMax=[]  SumI4OutMin=[]  SumI4OutMax=[]  SumDOutMin=[]  SumDOutMax=[]  DifferentiatorOutMin=[]  DifferentiatorOutMax=[]  FilterDiffOutCoefMin=[]  FilterDiffOutCoefMax=[]  ReciprocalOutMin=[]  ReciprocalOutMax=[]  SumDenOutMin=[]  SumDenOutMax=[]  SumNumOutMin=[]  SumNumOutMax=[]  DivideOutMin=[]  DivideOutMax=[]  UdiffTsProdOutMin=[]  UdiffTsProdOutMax=[]  NTsProdOutMin=[]  NTsProdOutMax=[]  UintegralTsProdOutMin=[]  UintegralTsProdOutMax=[]  UngainTsProdOutMin=[]  UngainTsProdOutMax=[]  ClampingZeroOutDataTypeStr=Inherit: Inherit via back propagation  ClampingZeroOutMin=[]  ClampingZeroOutMax=[]  FilterDenConstantOutDataTypeStr=Inherit: Inherit via back propagation  FilterDenConstantOutMin=[]  FilterDenConstantOutMax=[]  PCopyOutDataTypeStr=Inherit: Inherit via back propagation  PCopyOutMin=[]  PCopyOutMax=[]  NCopyOutDataTypeStr=Inherit: Inherit via back propagation  NCopyOutMin=[]  NCopyOutMax=[]  IntegratorContinuousStateAttributes=''  IntegratorStateMustResolveToSignalObject=off  IntegratorRTWStateStorageClass=Auto  FilterContinuousStateAttributes=''  FilterStateMustResolveToSignalObject=off  FilterRTWStateStorageClass=Auto  ParallelPVariant=InternalParameters  IdealPVariant=Disabled  IVariant=InternalParameters  DVariant=Disabled  IntegratorVariant=Discrete  SatVariant=Enabled  AWVariant=DiscClampingParallel  PCopyVariant=Disabled  TRVariant=Disabled  FdbkBlocksVariant=Forward  IdealPFdbkVariant=Disabled  SatFdbkVariant=Disabled  DerivativeFilterVariant=Disabled  NVariant=Disabled  NCopyVariant=Disabled_SignalSpec  FilterICVariant=Disabled  IntegratorICVariant=InternalICs  ExternalResetVariant=ExternalReset  TRSumVariant=Passthrough  SumFdbkVariant=Disabled  SumVariant=Sum_PI  TsampFilterVariant=InternalTs  TsampNgainVariant=Passthrough  TsampIntegralVariant=Disabled_SignalSpec  ExternalSaturationOutDataTypeStr=Inherit: Same as second input  DerivativeSourceVariant=Disabled  PreIntVariant=InternalPreInt
      settings: LibrarySourceBlock=mcbhdllib/Controls/Controllers/PI Controller
  Relay : Relay  OnSwitchValue=10  OffSwitchValue=1
  Subtract : Sum  Inputs=+-
  Dec_cmd : Outport
  wires:
  Vel_ref/1 -> Subtract/2
  Vel_fdk/1 -> Subtract/1
  PI Controller/1 -> Dec_cmd/1
  Subtract/1 -> PI Controller/1, Relay/1
  Relay/1 -> PI Controller/2

== system GVCU_HIL_simscape/Driver/Driver/LPF ==
  u : Inport
  Divide : Product  Inputs=/
  Error LPF : autolibutils/Cont LPF Dyn  aMode=aMode  dataType=off
  tauerr : Constant  Value=0.03  SampleTime=-1
  y : Outport  VectorParamsAs1DForOutWhenUnconnected=off
  wires:
  Error LPF/1 -> y/1
  Divide/1 -> Error LPF/2
  tauerr/1 -> Divide/1
  u/1 -> Error LPF/1

== system GVCU_HIL_simscape/GVCU - HiL/Commented messages/Message Output12 ==
  In1 : Inport
  Bus Selector : BusSelector  OutputSignals=e2e_alive_counter_disabled,e2e_checksum_disabled,e_motor_pump_fault,e_motor_pump_power_on,e_motor_pump_speed,e_motor_pump_warning,front_left_fan_fault,front_left_fan_power_on,front_left_fan_speed,front_left_fan_warning,hv_bat_pump_fault,hv_bat_pump_power_on,hv_bat_pump_speed,hv_bat_pump_warning
  S-Function_1 : S-Function  FunctionName=sigout  Parameters=dbName;nodeName;msgName;14;'e2e_alive_counter_disabled';'e2e_checksum_disabled';'e_motor_pump_fault';'e_motor_pump_power_on';'e_motor_pump_speed';'e_motor_pump_warning';'front_left_fan_fault';'front_left_fan_power_on';'front_left_fan_speed';'front_left_fan_warning';'hv_bat_pump_fault';'hv_bat_pump_power_on';'hv_bat_pump_speed';'hv_bat_pump_warning';VGetRawValueFlag(rawValue);'inherited'  SFunctionDeploymentMode=off  EnableBusSupport=off
      settings: AttributesFormatString=e2e_alive_counter_disabled\ne2e_checksum_disabled\ne_motor_pump_fault\ne_motor_pump_power_on\ne_motor_pump_speed\ne_motor_pump_warning\nfront_left_fan_fault\nfront_left_fan_power_on\nfront_left_fan_speed\nfront_left_fan_warning\nhv_bat_pump_fault\nhv_bat_pump_power_on\nhv_bat_pump_speed\nhv_bat_pump_warning\n
  wires:
  In1/1 -> Bus Selector/1
  Bus Selector/1 -> S-Function_1/1  "<e2e_alive_counter_disabled>"
  Bus Selector/2 -> S-Function_1/2  "<e2e_checksum_disabled>"
  Bus Selector/3 -> S-Function_1/3  "<e_motor_pump_fault>"
  Bus Selector/4 -> S-Function_1/4  "<e_motor_pump_power_on>"
  Bus Selector/5 -> S-Function_1/5  "<e_motor_pump_speed>"
  Bus Selector/6 -> S-Function_1/6  "<e_motor_pump_warning>"
  Bus Selector/7 -> S-Function_1/7  "<front_left_fan_fault>"
  Bus Selector/8 -> S-Function_1/8  "<front_left_fan_power_on>"
  Bus Selector/9 -> S-Function_1/9  "<front_left_fan_speed>"
  Bus Selector/10 -> S-Function_1/10  "<front_left_fan_warning>"
  Bus Selector/11 -> S-Function_1/11  "<hv_bat_pump_fault>"
  Bus Selector/12 -> S-Function_1/12  "<hv_bat_pump_power_on>"
  Bus Selector/13 -> S-Function_1/13  "<hv_bat_pump_speed>"
  Bus Selector/14 -> S-Function_1/14  "<hv_bat_pump_warning>"

== system GVCU_HIL_simscape/GVCU - HiL/Commented messages/Message Output13 ==
  In1 : Inport
  Bus Selector : BusSelector  OutputSignals=e2e_alive_counter_disabled,e2e_checksum_disabled,inverter_pump_fault,inverter_pump_power_on,inverter_pump_speed,inverter_pump_warning
  S-Function_1 : S-Function  FunctionName=sigout  Parameters=dbName;nodeName;msgName;6;'e2e_alive_counter_disabled';'e2e_checksum_disabled';'inverter_pump_fault';'inverter_pump_power_on';'inverter_pump_speed';'inverter_pump_warning';VGetRawValueFlag(rawValue);'inherited'  SFunctionDeploymentMode=off  EnableBusSupport=off
      settings: AttributesFormatString=e2e_alive_counter_disabled\ne2e_checksum_disabled\ninverter_pump_fault\ninverter_pump_power_on\ninverter_pump_speed\ninverter_pump_warning\n
  wires:
  In1/1 -> Bus Selector/1
  Bus Selector/1 -> S-Function_1/1  "<e2e_alive_counter_disabled>"
  Bus Selector/2 -> S-Function_1/2  "<e2e_checksum_disabled>"
  Bus Selector/3 -> S-Function_1/3  "<inverter_pump_fault>"
  Bus Selector/4 -> S-Function_1/4  "<inverter_pump_power_on>"
  Bus Selector/5 -> S-Function_1/5  "<inverter_pump_speed>"
  Bus Selector/6 -> S-Function_1/6  "<inverter_pump_warning>"

== system GVCU_HIL_simscape/GVCU - HiL/Commented messages/Message Output14 ==
  In1 : Inport
  Bus Selector : BusSelector  OutputSignals=u_lift_cyl_fl,u_lift_cyl_fr,u_wishbone_angle_fl,u_wishbone_angle_fr
  S-Function_1 : S-Function  FunctionName=sigout  Parameters=dbName;nodeName;msgName;4;'u_lift_cyl_fl';'u_lift_cyl_fr';'u_wishbone_angle_fl';'u_wishbone_angle_fr';VGetRawValueFlag(rawValue);'inherited'  SFunctionDeploymentMode=off  EnableBusSupport=off
      settings: AttributesFormatString=u_lift_cyl_fl\nu_lift_cyl_fr\nu_wishbone_angle_fl\nu_wishbone_angle_fr\n
  wires:
  In1/1 -> Bus Selector/1
  Bus Selector/1 -> S-Function_1/1  "<u_lift_cyl_fl>"
  Bus Selector/2 -> S-Function_1/2  "<u_lift_cyl_fr>"
  Bus Selector/3 -> S-Function_1/3  "<u_wishbone_angle_fl>"
  Bus Selector/4 -> S-Function_1/4  "<u_wishbone_angle_fr>"

== system GVCU_HIL_simscape/GVCU - HiL/Commented messages/Message Output15 ==
  In1 : Inport
  Bus Selector : BusSelector  OutputSignals=actv_re,snsr_data_rcl,snsr_data_rcr,snsr_data_rl,snsr_data_rll,snsr_data_rr,snsr_data_rrl,snsr_st_rcl,snsr_st_rcr,snsr_st_rl,snsr_st_rll,snsr_st_rr,snsr_st_rrl
  S-Function_1 : S-Function  FunctionName=sigout  Parameters=dbName;nodeName;msgName;13;'actv_re';'snsr_data_rcl';'snsr_data_rcr';'snsr_data_rl';'snsr_data_rll';'snsr_data_rr';'snsr_data_rrl';'snsr_st_rcl';'snsr_st_rcr';'snsr_st_rl';'snsr_st_rll';'snsr_st_rr';'snsr_st_rrl';VGetRawValueFlag(rawValue);'inherited'  SFunctionDeploymentMode=off  EnableBusSupport=off
      settings: AttributesFormatString=actv_re\nsnsr_data_rcl\nsnsr_data_rcr\nsnsr_data_rl\nsnsr_data_rll\nsnsr_data_rr\nsnsr_data_rrl\nsnsr_st_rcl\nsnsr_st_rcr\nsnsr_st_rl\nsnsr_st_rll\nsnsr_st_rr\nsnsr_st_rrl\n
  wires:
  In1/1 -> Bus Selector/1
  Bus Selector/1 -> S-Function_1/1  "<actv_re>"
  Bus Selector/2 -> S-Function_1/2  "<snsr_data_rcl>"
  Bus Selector/3 -> S-Function_1/3  "<snsr_data_rcr>"
  Bus Selector/4 -> S-Function_1/4  "<snsr_data_rl>"
  Bus Selector/5 -> S-Function_1/5  "<snsr_data_rll>"
  Bus Selector/6 -> S-Function_1/6  "<snsr_data_rr>"
  Bus Selector/7 -> S-Function_1/7  "<snsr_data_rrl>"
  Bus Selector/8 -> S-Function_1/8  "<snsr_st_rcl>"
  Bus Selector/9 -> S-Function_1/9  "<snsr_st_rcr>"
  Bus Selector/10 -> S-Function_1/10  "<snsr_st_rl>"
  Bus Selector/11 -> S-Function_1/11  "<snsr_st_rll>"
  Bus Selector/12 -> S-Function_1/12  "<snsr_st_rr>"
  Bus Selector/13 -> S-Function_1/13  "<snsr_st_rrl>"

== system GVCU_HIL_simscape/GVCU - HiL/Commented messages/Message Output16 ==
  In1 : Inport
  Bus Selector : BusSelector  OutputSignals=actv_frnt,snsr_data_fcl,snsr_data_fcr,snsr_data_fl,snsr_data_fll,snsr_data_fr,snsr_data_frl,snsr_st_fcl,snsr_st_fcr,snsr_st_fl,snsr_st_fll,snsr_st_fr,snsr_st_frl
  S-Function_1 : S-Function  FunctionName=sigout  Parameters=dbName;nodeName;msgName;13;'actv_frnt';'snsr_data_fcl';'snsr_data_fcr';'snsr_data_fl';'snsr_data_fll';'snsr_data_fr';'snsr_data_frl';'snsr_st_fcl';'snsr_st_fcr';'snsr_st_fl';'snsr_st_fll';'snsr_st_fr';'snsr_st_frl';VGetRawValueFlag(rawValue);'inherited'  SFunctionDeploymentMode=off  EnableBusSupport=off
      settings: AttributesFormatString=actv_frnt\nsnsr_data_fcl\nsnsr_data_fcr\nsnsr_data_fl\nsnsr_data_fll\nsnsr_data_fr\nsnsr_data_frl\nsnsr_st_fcl\nsnsr_st_fcr\nsnsr_st_fl\nsnsr_st_fll\nsnsr_st_fr\nsnsr_st_frl\n
  wires:
  In1/1 -> Bus Selector/1
  Bus Selector/1 -> S-Function_1/1  "<actv_frnt>"
  Bus Selector/2 -> S-Function_1/2  "<snsr_data_fcl>"
  Bus Selector/3 -> S-Function_1/3  "<snsr_data_fcr>"
  Bus Selector/4 -> S-Function_1/4  "<snsr_data_fl>"
  Bus Selector/5 -> S-Function_1/5  "<snsr_data_fll>"
  Bus Selector/6 -> S-Function_1/6  "<snsr_data_fr>"
  Bus Selector/7 -> S-Function_1/7  "<snsr_data_frl>"
  Bus Selector/8 -> S-Function_1/8  "<snsr_st_fcl>"
  Bus Selector/9 -> S-Function_1/9  "<snsr_st_fcr>"
  Bus Selector/10 -> S-Function_1/10  "<snsr_st_fl>"
  Bus Selector/11 -> S-Function_1/11  "<snsr_st_fll>"
  Bus Selector/12 -> S-Function_1/12  "<snsr_st_fr>"
  Bus Selector/13 -> S-Function_1/13  "<snsr_st_frl>"

== system GVCU_HIL_simscape/GVCU - HiL/Commented messages/Message Output2 ==
  In1 : Inport
  Bus Selector : BusSelector  OutputSignals=e2e_alive_counter_disabled,e2e_checksum_disabled,front_center_left_fan_fault,front_center_left_fan_power_on,front_center_left_fan_speed,front_center_left_fan_warning,front_center_right_fan_fault,front_center_right_fan_power_on,front_center_right_fan_speed,front_center_right_fan_warning,front_right_fan_fault,front_right_fan_power_on,front_right_fan_speed,front_right_fan_warning
  S-Function_1 : S-Function  FunctionName=sigout  Parameters=dbName;nodeName;msgName;14;'e2e_alive_counter_disabled';'e2e_checksum_disabled';'front_center_left_fan_fault';'front_center_left_fan_power_on';'front_center_left_fan_speed';'front_center_left_fan_warning';'front_center_right_fan_fault';'front_center_right_fan_power_on';'front_center_right_fan_speed';'front_center_right_fan_warning';'front_right_fan_fault';'front_right_fan_power_on';'front_right_fan_speed';'front_right_fan_warning';VGetRawValueFlag(rawValue);'inherited'  SFunctionDeploymentMode=off  EnableBusSupport=off
      settings: AttributesFormatString=e2e_alive_counter_disabled\ne2e_checksum_disabled\nfront_center_left_fan_fault\nfront_center_left_fan_power_on\nfront_center_left_fan_speed\nfront_center_left_fan_warning\nfront_center_right_fan_fault\nfront_center_right_fan_power_on\nfront_center_right_fan_speed\nfront_center_right_fan_warning\nfront_right_fan_fault\nfront_right_fan_power_on\nfront_right_fan_speed\nfront_right_fan_warning\n
  wires:
  In1/1 -> Bus Selector/1
  Bus Selector/1 -> S-Function_1/1  "<e2e_alive_counter_disabled>"
  Bus Selector/2 -> S-Function_1/2  "<e2e_checksum_disabled>"
  Bus Selector/3 -> S-Function_1/3  "<front_center_left_fan_fault>"
  Bus Selector/4 -> S-Function_1/4  "<front_center_left_fan_power_on>"
  Bus Selector/5 -> S-Function_1/5  "<front_center_left_fan_speed>"
  Bus Selector/6 -> S-Function_1/6  "<front_center_left_fan_warning>"
  Bus Selector/7 -> S-Function_1/7  "<front_center_right_fan_fault>"
  Bus Selector/8 -> S-Function_1/8  "<front_center_right_fan_power_on>"
  Bus Selector/9 -> S-Function_1/9  "<front_center_right_fan_speed>"
  Bus Selector/10 -> S-Function_1/10  "<front_center_right_fan_warning>"
  Bus Selector/11 -> S-Function_1/11  "<front_right_fan_fault>"
  Bus Selector/12 -> S-Function_1/12  "<front_right_fan_power_on>"
  Bus Selector/13 -> S-Function_1/13  "<front_right_fan_speed>"
  Bus Selector/14 -> S-Function_1/14  "<front_right_fan_warning>"

== system GVCU_HIL_simscape/GVCU - HiL/Commented messages/Message Output20 ==
  In1 : Inport
  Bus Selector : BusSelector  OutputSignals=E2eAliveCounter_Disable,E2eChecksum_Disable,acc_dft_actv_st,acc_dft_dist_lvl,auto_upsh_btn_st,drv_cfg_req,drv_st,esp_st_req,forced_chrg_btn_st,lift_mod_btn_st,man_mod_btn_st,suppg_mod_req,tire_mdl_req
  S-Function_1 : S-Function  FunctionName=sigout  Parameters=dbName;nodeName;msgName;13;'E2eAliveCounter_Disable';'E2eChecksum_Disable';'acc_dft_actv_st';'acc_dft_dist_lvl';'auto_upsh_btn_st';'drv_cfg_req';'drv_mod_req';'esp_st_req';'forced_chrg_btn_st';'lift_mod_btn_st';'man_mod_btn_st';'suppg_mod_req';'tire_mdl_req';VGetRawValueFlag(rawValue);'inherited'  SFunctionDeploymentMode=off  EnableBusSupport=off
      settings: AttributesFormatString=E2eAliveCounter_Disable\nE2eChecksum_Disable\nacc_dft_actv_st\nacc_dft_dist_lvl\nauto_upsh_btn_st\ndrv_cfg_req\ndrv_mod_req\nesp_st_req\nforced_chrg_btn_st\nlift_mod_btn_st\nman_mod_btn_st\nsuppg_mod_req\ntire_mdl_req\n
  wires:
  In1/1 -> Bus Selector/1
  Bus Selector/1 -> S-Function_1/1  "<E2eAliveCounter_Disable>"
  Bus Selector/2 -> S-Function_1/2  "<E2eChecksum_Disable>"
  Bus Selector/3 -> S-Function_1/3  "<acc_dft_actv_st>"
  Bus Selector/4 -> S-Function_1/4  "<acc_dft_dist_lvl>"
  Bus Selector/5 -> S-Function_1/5  "<auto_upsh_btn_st>"
  ? -> S-Function_1/6  "<drift_mod_st_req>"
  Bus Selector/6 -> S-Function_1/7  "<drv_cfg_req>"
  Bus Selector/7 -> S-Function_1/8  "<drv_st>"
  Bus Selector/8 -> S-Function_1/9  "<esp_st_req>"
  Bus Selector/9 -> S-Function_1/10  "<forced_chrg_btn_st>"
  Bus Selector/10 -> S-Function_1/11  "<lift_mod_btn_st>"
  Bus Selector/11 -> S-Function_1/12  "<man_mod_btn_st>"
  Bus Selector/13 -> S-Function_1/13  "<tire_mdl_req>"

== system GVCU_HIL_simscape/GVCU - HiL/Commented messages/Message Output4 ==
  In1 : Inport
  Bus Selector : BusSelector  OutputSignals=CrashSeverity,DriverSideCrash,E2eAliveCounter,E2eChecksum,FrontCrash,PassSideCrash,RearCrash,RolloverCrash
  S-Function_1 : S-Function  FunctionName=sigout  Parameters=dbName;nodeName;msgName;8;'CrashSeverity';'DriverSideCrash';'E2eAliveCounter';'E2eChecksum';'FrontCrash';'PassSideCrash';'RearCrash';'RolloverCrash';VGetRawValueFlag(rawValue);'inherited'  SFunctionDeploymentMode=off  EnableBusSupport=off
      settings: AttributesFormatString=CrashSeverity\nDriverSideCrash\nE2eAliveCounter\nE2eChecksum\nFrontCrash\nPassSideCrash\nRearCrash\nRolloverCrash\n
  wires:
  In1/1 -> Bus Selector/1
  Bus Selector/1 -> S-Function_1/1  "<CrashSeverity>"
  Bus Selector/2 -> S-Function_1/2  "<DriverSideCrash>"
  Bus Selector/3 -> S-Function_1/3  "<E2eAliveCounter>"
  Bus Selector/4 -> S-Function_1/4  "<E2eChecksum>"
  Bus Selector/5 -> S-Function_1/5  "<FrontCrash>"
  Bus Selector/6 -> S-Function_1/6  "<PassSideCrash>"
  Bus Selector/7 -> S-Function_1/7  "<RearCrash>"
  Bus Selector/8 -> S-Function_1/8  "<RolloverCrash>"

== system GVCU_HIL_simscape/GVCU - HiL/Commented messages/Message Output5 ==
  In1 : Inport
  Bus Selector : BusSelector  OutputSignals=CrashOutput,E2eAliveCounter,E2eChecksum
  S-Function_1 : S-Function  FunctionName=sigout  Parameters=dbName;nodeName;msgName;3;'CrashOutput';'E2eAliveCounter';'E2eChecksum';VGetRawValueFlag(rawValue);'inherited'  SFunctionDeploymentMode=off  EnableBusSupport=off
      settings: AttributesFormatString=CrashOutput\nE2eAliveCounter\nE2eChecksum\n
  wires:
  In1/1 -> Bus Selector/1
  Bus Selector/1 -> S-Function_1/1  "<CrashOutput>"
  Bus Selector/2 -> S-Function_1/2  "<E2eAliveCounter>"
  Bus Selector/3 -> S-Function_1/3  "<E2eChecksum>"

== system GVCU_HIL_simscape/GVCU - HiL/Commented messages/Message Output6 ==
  In1 : Inport
  Bus Selector : BusSelector  OutputSignals=center_left_fan_bat_vltg,center_left_fan_can_collision,center_left_fan_can_watchdog,center_left_fan_motor_stall,center_left_fan_over_crnt,center_left_fan_over_pwr,center_left_fan_over_temp,center_right_fan_bat_vltg,center_right_fan_can_collision,center_right_fan_can_watchdog,center_right_fan_motor_stall,center_right_fan_over_crnt,center_right_fan_over_pwr,center_right_fan_over_temp,e_mot_pump_comm_fault,e_mot_pump_int_op_fault,e_mot_pump_over_crnt,e_mot_pump_over_temp,e_mot_pump_vltg_err,front_left_fan_bat_vltg,front_left_fan_can_collision,front_left_fan_can_watchdog,front_left_fan_motor_stall,front_left_fan_over_crnt,front_left_fan_over_pwr,front_left_fan_over_temp,front_right_fan_bat_vltg,front_right_fan_can_collision,front_right_fan_can_watchdog,front_right_fan_motor_stall,front_right_fan_over_crnt,front_right_fan_over_pwr,front_right_fan_over_temp,hv_bat_pump_bat_vltg,hv_bat_pump_can_collision,hv_bat_pump_can_watchdog,hv_bat_pump_motor_stall,hv_bat_pump_over_crnt,hv_bat_pump_over_pwr,hv_bat_pump_over_temp,inverter_pump_bat_vltg,inverter_pump_can_collision,inverter_pump_can_watchdog,inverter_pump_motor_stall,inverter_pump_over_crnt,inverter_pump_over_pwr,inverter_pump_over_temp
  S-Function_1 : S-Function  FunctionName=sigout  Parameters=dbName;nodeName;msgName;47;'center_left_fan_bat_vltg';'center_left_fan_can_collision';'center_left_fan_can_watchdog';'center_left_fan_motor_stall';'center_left_fan_over_crnt';'center_left_fan_over_pwr';'center_left_fan_over_temp';'center_right_fan_bat_vltg';'center_right_fan_can_collision';'center_right_fan_can_watchdog';'center_right_fan_motor_stall';'center_right_fan_over_crnt';'center_right_fan_over_pwr';'center_right_fan_over_temp';'e_mot_pump_comm_fault';'e_mot_pump_int_op_fault';'e_mot_pump_over_crnt';'e_mot_pump_over_temp';'e_mot_pump_vltg_err';'front_left_fan_bat_vltg';'front_left_fan_can_collision';'front_left_fan_can_watchdog';'front_left_fan_motor_stall';'front_left_fan_over_crnt';'front_left_fan_over_pwr';'front_left_fan_over_temp';'front_right_fan_bat_vltg';'front_right_fan_can_collision';'front_right_fan_can_watchdog';'front_right_fan_motor_stall';'front_right_fan_over_crnt';'front_right_fan_over_pwr';'front_right_fan_over_temp';'hv_bat_pump_bat_vltg';'hv_bat_pump_can_collision';'hv_bat_pump_can_watchdog';'hv_bat_pump_motor_stall';'hv_bat_pump_over_crnt';'hv_bat_pump_over_pwr';'hv_bat_pump_over_temp';'inverter_pump_bat_vltg';'inverter_pump_can_collision';'inverter_pump_can_watchdog';'inverter_pump_motor_stall';'inverter_pump_over_crnt';'inverter_pump_over_pwr';'inverter_pump_over_temp';VGetRawValueFlag(rawValue);'inherited'  SFunctionDeploymentMode=off  EnableBusSupport=off
      settings: AttributesFormatString=center_left_fan_bat_vltg\ncenter_left_fan_can_collision\ncenter_left_fan_can_watchdog\ncenter_left_fan_motor_stall\ncenter_left_fan_over_crnt\ncenter_left_fan_over_pwr\ncenter_left_fan_over_temp\ncenter_right_fan_bat_vltg\ncenter_right_fan_can_collision\ncenter_right_fan_can_watchdog\ncenter_right_fan_motor_stall\ncenter_right_fan_over_crnt\ncenter_right_fan_over_pwr\ncenter_right_fan_over_temp\ne_mot_pump_comm_fault\ne_mot_pump_int_op_fault\ne_mot_pump_over_crnt\ne_mot_pump_over_temp\ne_mot_pump_vltg_err\nfront_left_fan_bat_vltg\nfront_left_fan_can_collision\nfront_left_fan_can_watchdog\nfront_left_fan_motor_stall\nfront_left_fan_over_crnt\nfront_left_fan_over_pwr\nfront_left_fan_over_temp\nfront_right_fan_bat_vltg\nfront_right_fan_can_collision\nfront_right_fan_can_watchdog\nfront_right_fan_motor_stall\nfront_right_fan_over_crnt\nfront_right_fan_over_pwr\nfront_right_fan_over_temp\nhv_bat_pump_bat_vltg\nhv_bat_pump_can_collision\nhv_bat_pump_can_watchdog\nhv_bat_pump_motor_stall\nhv_bat_pump_over_crnt\nhv_bat_pump_over_pwr\nhv_bat_pump_over_temp\ninverter_pump_bat_vltg\ninverter_pump_can_collision\ninverter_pump_can_watchdog\ninverter_pump_motor_stall\ninverter_pump_over_crnt\ninverter_pump_over_pwr\ninverter_pump_over_temp\n
  wires:
  In1/1 -> Bus Selector/1
  Bus Selector/1 -> S-Function_1/1  "<center_left_fan_bat_vltg>"
  Bus Selector/2 -> S-Function_1/2  "<center_left_fan_can_collision>"
  Bus Selector/3 -> S-Function_1/3  "<center_left_fan_can_watchdog>"
  Bus Selector/4 -> S-Function_1/4  "<center_left_fan_motor_stall>"
  Bus Selector/5 -> S-Function_1/5  "<center_left_fan_over_crnt>"
  Bus Selector/6 -> S-Function_1/6  "<center_left_fan_over_pwr>"
  Bus Selector/7 -> S-Function_1/7  "<center_left_fan_over_temp>"
  Bus Selector/8 -> S-Function_1/8  "<center_right_fan_bat_vltg>"
  Bus Selector/9 -> S-Function_1/9  "<center_right_fan_can_collision>"
  Bus Selector/10 -> S-Function_1/10  "<center_right_fan_can_watchdog>"
  Bus Selector/11 -> S-Function_1/11  "<center_right_fan_motor_stall>"
  Bus Selector/12 -> S-Function_1/12  "<center_right_fan_over_crnt>"
  Bus Selector/13 -> S-Function_1/13  "<center_right_fan_over_pwr>"
  Bus Selector/14 -> S-Function_1/14  "<center_right_fan_over_temp>"
  Bus Selector/15 -> S-Function_1/15  "<e_mot_pump_comm_fault>"
  Bus Selector/16 -> S-Function_1/16  "<e_mot_pump_int_op_fault>"
  Bus Selector/17 -> S-Function_1/17  "<e_mot_pump_over_crnt>"
  Bus Selector/18 -> S-Function_1/18  "<e_mot_pump_over_temp>"
  Bus Selector/19 -> S-Function_1/19  "<e_mot_pump_vltg_err>"
  Bus Selector/20 -> S-Function_1/20  "<front_left_fan_bat_vltg>"
  Bus Selector/21 -> S-Function_1/21  "<front_left_fan_can_collision>"
  Bus Selector/22 -> S-Function_1/22  "<front_left_fan_can_watchdog>"
  Bus Selector/23 -> S-Function_1/23  "<front_left_fan_motor_stall>"
  Bus Selector/24 -> S-Function_1/24  "<front_left_fan_over_crnt>"
  Bus Selector/25 -> S-Function_1/25  "<front_left_fan_over_pwr>"
  Bus Selector/26 -> S-Function_1/26  "<front_left_fan_over_temp>"
  Bus Selector/27 -> S-Function_1/27  "<front_right_fan_bat_vltg>"
  Bus Selector/28 -> S-Function_1/28  "<front_right_fan_can_collision>"
  Bus Selector/29 -> S-Function_1/29  "<front_right_fan_can_watchdog>"
  Bus Selector/30 -> S-Function_1/30  "<front_right_fan_motor_stall>"
  Bus Selector/31 -> S-Function_1/31  "<front_right_fan_over_crnt>"
  Bus Selector/32 -> S-Function_1/32  "<front_right_fan_over_pwr>"
  Bus Selector/33 -> S-Function_1/33  "<front_right_fan_over_temp>"
  Bus Selector/34 -> S-Function_1/34  "<hv_bat_pump_bat_vltg>"
  Bus Selector/35 -> S-Function_1/35  "<hv_bat_pump_can_collision>"
  Bus Selector/36 -> S-Function_1/36  "<hv_bat_pump_can_watchdog>"
  Bus Selector/37 -> S-Function_1/37  "<hv_bat_pump_motor_stall>"
  Bus Selector/38 -> S-Function_1/38  "<hv_bat_pump_over_crnt>"
  Bus Selector/39 -> S-Function_1/39  "<hv_bat_pump_over_pwr>"
  Bus Selector/40 -> S-Function_1/40  "<hv_bat_pump_over_temp>"
  Bus Selector/41 -> S-Function_1/41  "<inverter_pump_bat_vltg>"
  Bus Selector/42 -> S-Function_1/42  "<inverter_pump_can_collision>"
  Bus Selector/43 -> S-Function_1/43  "<inverter_pump_can_watchdog>"
  Bus Selector/44 -> S-Function_1/44  "<inverter_pump_motor_stall>"
  Bus Selector/45 -> S-Function_1/45  "<inverter_pump_over_crnt>"
  Bus Selector/46 -> S-Function_1/46  "<inverter_pump_over_pwr>"
  Bus Selector/47 -> S-Function_1/47  "<inverter_pump_over_temp>"
